simulink model "qudorsey"  (R2025b)
settings: Solver=ode113  StartTime=0.0  StopTime=100.0  RelTol=1e-10
values from neighbouring files (symbols this model uses):
  A = 7    [qudorsey_init.m]
  B = 8    [qudorsey_init.m]
  C = 1    [qudorsey_init.m]
  D = 7    [qudorsey_init.m]
  g = 9.81    [qudorsey_init.m]
  Kd = [Kd11 0; 0 Kd11]    [qudorsey_init.m]
  Kp = [Kp11 0; 0 Kp11]    [qudorsey_init.m]
  theta1 = 3.1    [qudorsey_init.m]
  theta2 = 9.5    [qudorsey_init.m]
  theta3 = 0.24    [qudorsey_init.m]
  theta4 = 0.77    [qudorsey_init.m]
settings Model: Creator=cardaver  LastModifiedBy=cardaver

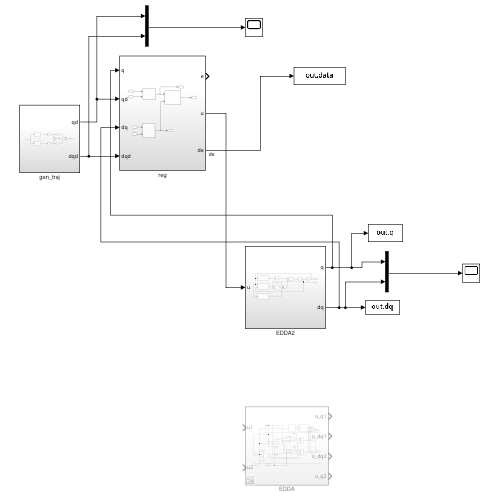
[thumbnail: Simulink's stored preview of the top-level diagram]
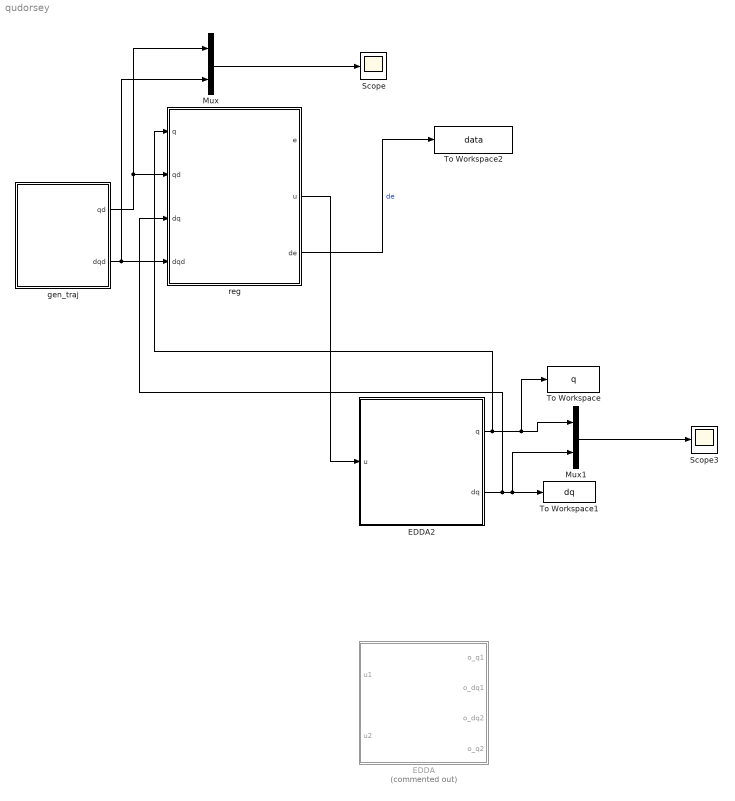
== system qudorsey ==
  EDDA : Subsystem  Commented=on
  EDDA2 : Subsystem
  Mux : Mux  Inputs=2
  Mux1 : Mux  Inputs=2
  Scope : Scope
      settings: ActiveDisplayYMinimum=-8.74999999993033  ActiveDisplayYMaximum=8.7499999999922586
  Scope3 : Scope
      settings: ActiveDisplayYMinimum=-60.558319819676356  ActiveDisplayYMaximum=101.0495694781887  DataLoggingVariableName=ScopeData3
  To Workspace : ToWorkspace  VariableName=q  SampleTime=-1
      settings: Save2DSignal=2-D array (concatenate along first dimension)
  To Workspace1 : ToWorkspace  VariableName=dq  SampleTime=-1
      settings: Save2DSignal=2-D array (concatenate along first dimension)
  To Workspace2 : ToWorkspace  VariableName=data  SaveFormat=Timeseries  SampleTime=-1
  gen_traj : Subsystem
  reg : Subsystem
  wires:
  EDDA2/1(q) -> Mux1/1, To Workspace/1, reg/1(q)
  Mux/1 -> Scope/1
  EDDA2/2(dq) -> To Workspace1/1, Mux1/2, reg/3(dq)
  gen_traj/1(qd) -> reg/2(qd), Mux/1
  gen_traj/2(dqd) -> reg/4(dqd), Mux/2
  Mux1/1 -> Scope3/1
  reg/2(u) -> EDDA2/1(u)
  reg/3(de) -> To Workspace2/1  "de"

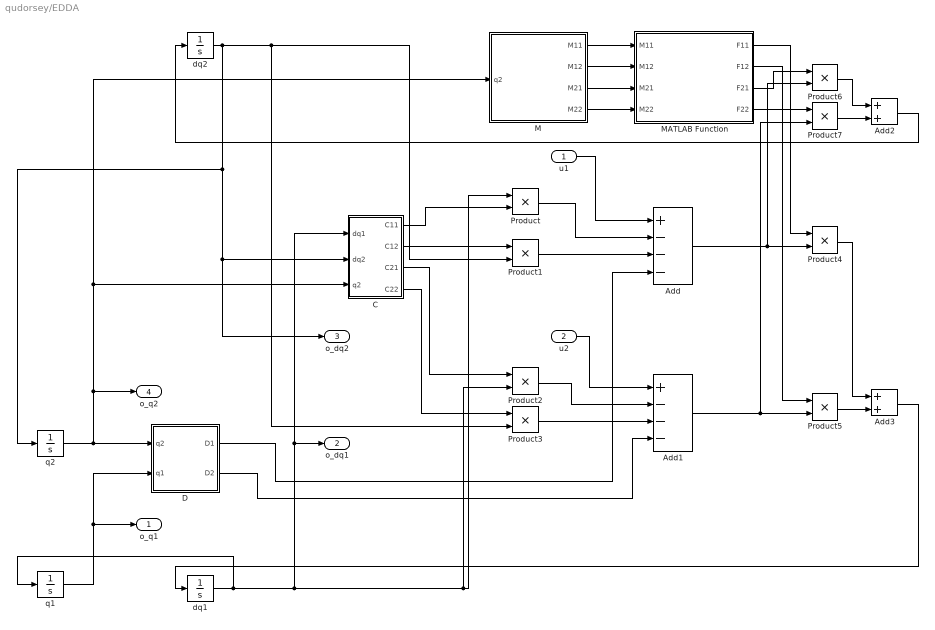
== system qudorsey/EDDA ==
  u1 : Inport
  u2 : Inport  Port=2
  Add : Sum  Inputs=+---
  Add1 : Sum  Inputs=+---
  Add2 : Sum
  Add3 : Sum
  C : Subsystem
  D : Subsystem
  M : Subsystem
  MATLAB Function : MATLAB Function  TreatAsAtomicUnit=on
  Product{,1..7} (8 alike) : Product
  dq1 : Integrator
  dq2 : Integrator
  q1 : Integrator
  q2 : Integrator
  o_q1 : Outport
  o_dq1 : Outport  Port=2
  o_dq2 : Outport  Port=3
  o_q2 : Outport  Port=4
  wires:
  D/2(D2) -> Add1/4
  C/3(C21) -> Product2/1
  u1/1 -> Add/1
  M/3(M21) -> MATLAB Function/3(M21)
  Add3/1 -> dq1/1
  MATLAB Function/3(F21) -> Product6/1
  q1/1 -> o_q1/1, D/2(q1)
  Add/1 -> Product6/2, Product4/2
  Product7/1 -> Add2/2
  dq1/1 -> Product2/2, Product/1, o_dq1/1, C/1(dq1), q1/1
  u2/1 -> Add1/1
  MATLAB Function/2(F12) -> Product5/1
  C/2(C12) -> Product1/1
  q2/1 -> o_q2/1, C/3(q2), M/1(q2), D/1(q2)
  dq2/1 -> o_dq2/1, C/2(dq2), q2/1, Product3/2, Product1/2
  M/2(M12) -> MATLAB Function/2(M12)
  M/4(M22) -> MATLAB Function/4(M22)
  Product4/1 -> Add3/1
  C/1(C11) -> Product/2
  M/1(M11) -> MATLAB Function/1(M11)
  MATLAB Function/4(F22) -> Product7/1
  Product1/1 -> Add/3
  C/4(C22) -> Product3/1
  Add1/1 -> Product7/2, Product5/2
  Add2/1 -> dq2/1
  Product3/1 -> Add1/3
  Product/1 -> Add/2
  Product5/1 -> Add3/2
  MATLAB Function/1(F11) -> Product4/1
  D/1(D1) -> Add/4
  Product2/1 -> Add1/2
  Product6/1 -> Add2/1

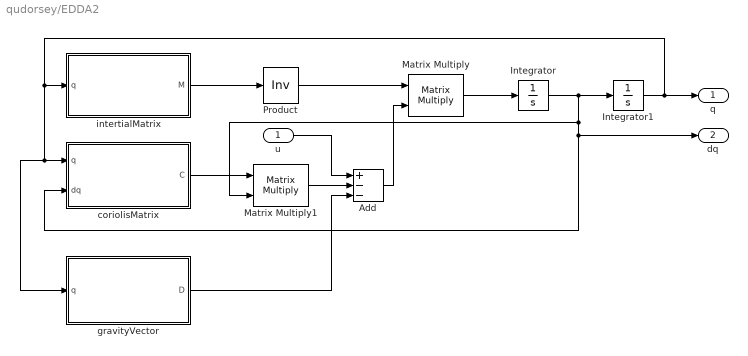
== system qudorsey/EDDA2 ==
  u : Inport
  Add : Sum  Inputs=+--
  Integrator : Integrator  InitialCondition=zeros(2,1)
  Integrator1 : Integrator  InitialCondition=[0;0]
  Matrix Multiply : Product  Multiplication=Matrix(*)
  Matrix Multiply1 : Product  Multiplication=Matrix(*)
  Product : Product  Inputs=/  Multiplication=Matrix(*)
  coriolisMatrix : MATLAB Function  TreatAsAtomicUnit=on
  gravityVector : MATLAB Function  TreatAsAtomicUnit=on
  intertialMatrix : MATLAB Function  TreatAsAtomicUnit=on
  q : Outport  PortDimensions=2
  dq : Outport  Port=2  PortDimensions=2
  wires:
  Product/1 -> Matrix Multiply/1
  gravityVector/1(D) -> Add/3
  Integrator/1 -> dq/1, coriolisMatrix/2(dq), Matrix Multiply1/2, Integrator1/1
  Matrix Multiply/1 -> Integrator/1
  Add/1 -> Matrix Multiply/2
  Integrator1/1 -> q/1, coriolisMatrix/1(q), gravityVector/1(q), intertialMatrix/1(q)
  intertialMatrix/1(M) -> Product/1
  coriolisMatrix/1(C) -> Matrix Multiply1/1
  Matrix Multiply1/1 -> Add/2
  u/1 -> Add/1

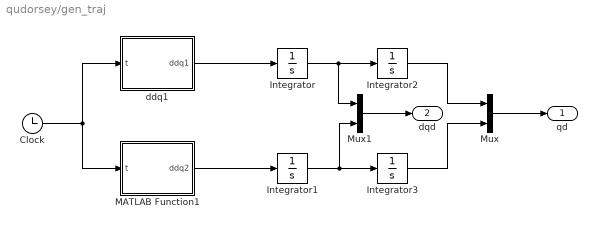
== system qudorsey/gen_traj ==
  Clock : Clock
  Integrator : Integrator
  Integrator1 : Integrator  InitialCondition=C/D
  Integrator2 : Integrator  InitialCondition=A
  Integrator3 : Integrator
  MATLAB Function1 : MATLAB Function  TreatAsAtomicUnit=on
  Mux : Mux  Inputs=2
  Mux1 : Mux  Inputs=2
  ddq1 : MATLAB Function  TreatAsAtomicUnit=on
  qd : Outport
  dqd : Outport  Port=2
  wires:
  Integrator1/1 -> Mux1/2, Integrator3/1
  Integrator3/1 -> Mux/2
  Integrator/1 -> Mux1/1, Integrator2/1
  ddq1/1(ddq1) -> Integrator/1
  Integrator2/1 -> Mux/1
  MATLAB Function1/1(ddq2) -> Integrator1/1
  Mux/1 -> qd/1
  Clock/1 -> MATLAB Function1/1(t), ddq1/1(t)
  Mux1/1 -> dqd/1

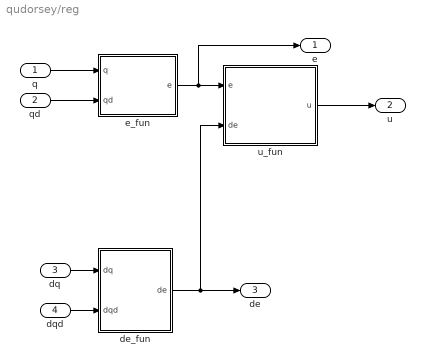
== system qudorsey/reg ==
  q : Inport
  qd : Inport  Port=2
  dq : Inport  Port=3
  dqd : Inport  Port=4
  de_fun : MATLAB Function  TreatAsAtomicUnit=on
  e_fun : MATLAB Function  TreatAsAtomicUnit=on
  u_fun : MATLAB Function  TreatAsAtomicUnit=on
  e : Outport
  u : Outport  Port=2
  de : Outport  Port=3
  wires:
  u_fun/1(u) -> u/1
  e_fun/1(e) -> e/1, u_fun/1(e)
  dq/1 -> de_fun/1(dq)
  q/1 -> e_fun/1(q)
  qd/1 -> e_fun/2(qd)
  dqd/1 -> de_fun/2(dqd)
  de_fun/1(de) -> de/1, u_fun/2(de)

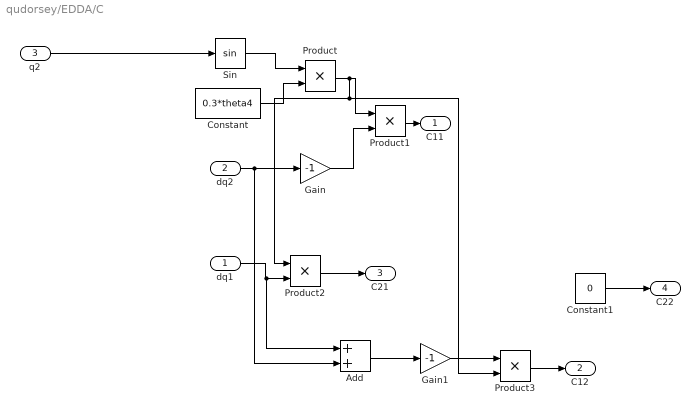
== system qudorsey/EDDA/C ==
  dq1 : Inport
  dq2 : Inport  Port=2
  q2 : Inport  Port=3
  Add : Sum
  Constant : Constant  Value=0.3*theta4
  Constant1 : Constant  Value=0
  Gain : Gain  Gain=-1
  Gain1 : Gain  Gain=-1
  Product{,1..3} (4 alike) : Product
  Sin : Trigonometry
  C11 : Outport
  C12 : Outport  Port=2
  C21 : Outport  Port=3
  C22 : Outport  Port=4
  wires:
  Sin/1 -> Product/1
  Constant/1 -> Product/2
  q2/1 -> Sin/1
  dq2/1 -> Add/2, Gain/1
  Product/1 -> Product2/1, Product3/2, Product1/1
  Gain/1 -> Product1/2
  Product1/1 -> C11/1
  dq1/1 -> Add/1, Product2/2
  Product2/1 -> C21/1
  Constant1/1 -> C22/1
  Add/1 -> Gain1/1
  Gain1/1 -> Product3/1
  Product3/1 -> C12/1

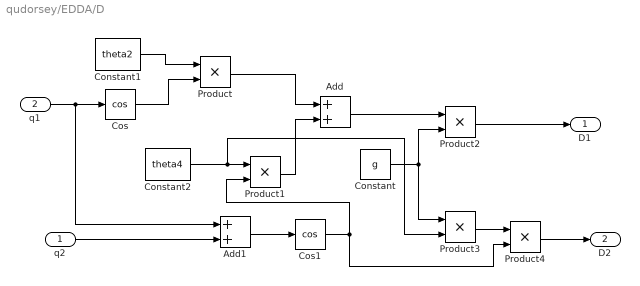
== system qudorsey/EDDA/D ==
  q2 : Inport
  q1 : Inport  Port=2
  Add : Sum
  Add1 : Sum
  Constant : Constant  Value=g
  Constant1 : Constant  Value=theta2
  Constant2 : Constant  Value=theta4
  Cos : Trigonometry  Operator=cos
  Cos1 : Trigonometry  Operator=cos
  Product{,1..4} (5 alike) : Product
  D1 : Outport
  D2 : Outport  Port=2
  wires:
  Product/1 -> Add/1
  q2/1 -> Add1/2
  Constant/1 -> Product3/1, Product2/2
  Add1/1 -> Cos1/1
  Constant1/1 -> Product/1
  Product3/1 -> Product4/1
  Product4/1 -> D2/1
  Cos1/1 -> Product4/2, Product1/2
  Constant2/1 -> Product3/2, Product1/1
  q1/1 -> Add1/1, Cos/1
  Product1/1 -> Add/2
  Add/1 -> Product2/1
  Product2/1 -> D1/1
  Cos/1 -> Product/2

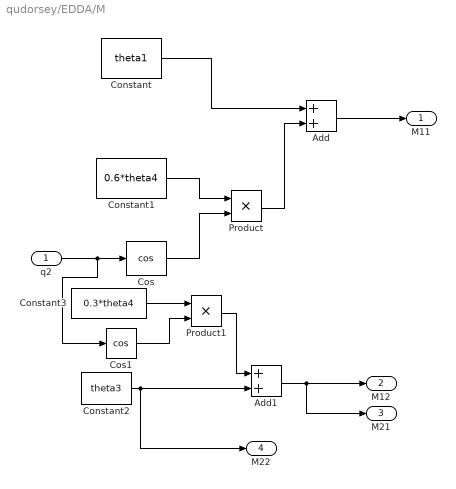
== system qudorsey/EDDA/M ==
  q2 : Inport
  Add : Sum
  Add1 : Sum
  Constant : Constant  Value=theta1
  Constant1 : Constant  Value=0.6*theta4
  Constant2 : Constant  Value=theta3
  Constant3 : Constant  Value=0.3*theta4
  Cos : Trigonometry  Operator=cos
  Cos1 : Trigonometry  Operator=cos
  Product : Product
  Product1 : Product
  M11 : Outport
  M12 : Outport  Port=2
  M21 : Outport  Port=3
  M22 : Outport  Port=4
  wires:
  Product/1 -> Add/2
  Constant3/1 -> Product1/1
  Add1/1 -> M12/1, M21/1
  Constant1/1 -> Product/1
  Cos/1 -> Product/2
  q2/1 -> Cos1/1, Cos/1
  Constant/1 -> Add/1
  Add/1 -> M11/1
  Product1/1 -> Add1/1
  Cos1/1 -> Product1/2
  Constant2/1 -> M22/1, Add1/2

== matlab function qudorsey/gen_traj/ddq1 ==
  data: t input; ddq1 output; A parameter; B parameter
function ddq1 = fcn(t, A, B)

ddq1 = (-A/(B^2))*cos(t/B);

== matlab function qudorsey/EDDA/MATLAB Function ==
  data: M11 input; F11 output; M12 input; M21 input; M22 input; F12 output; F21 output; F22 output
function [F11, F12, F21, F22] = INV(M11, M12, M21, M22)
    M = [M11, M12, M21, M22];
    M_inv = inv(M);
    
    F11 = M_inv(:, 1);
    F12 = M_inv(:, 2);
    F21 = M_inv(:, 3);
    F22 = M_inv(:, 4);
end

== matlab function qudorsey/gen_traj/MATLAB Function1 ==
  data: t input; ddq2 output; C parameter; D parameter
function ddq2 = fcn(t, C, D)

ddq2 = -(C^2/D)*sin(C*t);

== matlab function qudorsey/reg/e_fun ==
  data: q input; e output; qd input
function e = fcn(q, qd)

e = q - qd;

== matlab function qudorsey/reg/u_fun ==
  data: e input; u output; de input; Kp parameter; Kd parameter
function u = fcn(e, de, Kp, Kd)

u = -(Kp*e)-(Kd*de);

== matlab function qudorsey/reg/de_fun ==
  data: dq input; de output; dqd input
function de = fcn(dq, dqd)

de = dq - dqd;

== matlab function qudorsey/EDDA2/intertialMatrix ==
  data: M output; q input; theta1 parameter; theta4 parameter; theta3 parameter
function M = fcn(q, theta1, theta4, theta3)

q2 = q(2);

M = [theta1 + 0.6*theta4*cos(q2), theta3+0.3*theta4*cos(q2);
    theta3+0.3*theta4*cos(q2), theta3];

== matlab function qudorsey/EDDA2/coriolisMatrix ==
  data: q input; C output; dq input; theta4 parameter
function C = coriolisMatrix(q, dq, theta4)

q2 = q(2);
dq1 = dq(1);
dq2 = dq(2);

C = [-dq2, -(dq1 + dq2); dq1, 0]*0.3*theta4*sin(q2);

== matlab function qudorsey/EDDA2/gravityVector ==
  data: D output; q input; theta2 parameter; g parameter; theta4 parameter
function D = fcn(q, theta2, g, theta4)

q1 = q(1);
q2 = q(2);

D = g*[theta2*cos(q1) + theta4*cos(q1+q2);
    theta4*cos(q1+q2)];
